simulink library "cdsEpicsInCtrl"  (Simulink 7.2)
settings: Solver=ode45  SolverMode=SingleTasking  StartTime=0.0  StopTime=10.0  RelTol=1e-3
settings Model: Creator=maronsso  LastModifiedBy=aivanov

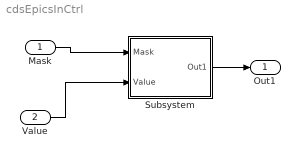
== system cdsEpicsInCtrl ==
  Mask : Inport  OutDataType=sfix(16)  OutScaling=2^0
  Value : Inport  Port=2  OutDataType=sfix(16)  OutScaling=2^0
  Subsystem : Subsystem  Tag=cdsEpicsInCtrl  Description=|
      | Purpose:                                                                                                                               
      | Create an EPICS input channel connection to the FE realtime controls. Allow                                                            
      | FE to control the value if Mask input is set to 1, in which case the value becomes                                                     
      | really the output value and treated by the EPICS CA as read only.                                                                      
      |                                                                                                                                        
      | Operation:                                                                                                                             
      | Outputs value from an EPICS ai record. Value is floating point with a precision of 3. Takes the mask and the values inputs from the FE.
      | Usage:                                                                                                                                 
      | Name the part with the desired EPICS channel name.
      settings: AttributesFormatString=%<Tag>
  Out1 : Outport  OutDataType=sfix(16)  OutScaling=2^0
  wires:
  Subsystem/1(Out1) -> Out1/1
  Value/1 -> Subsystem/2(Value)
  Mask/1 -> Subsystem/1(Mask)

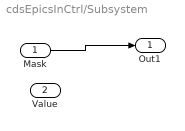
== system cdsEpicsInCtrl/Subsystem ==
  Mask : Inport  OutDataType=sfix(16)  OutScaling=2^0
  Value : Inport  Port=2  OutDataType=sfix(16)  OutScaling=2^0
  Out1 : Outport  OutDataType=sfix(16)  OutScaling=2^0
  wires:
  Mask/1 -> Out1/1
